simulink model "test"  (R2018b)
settings: Solver=VariableStepAuto  StartTime=0.0  StopTime=10  RelTol=1e-3
values from neighbouring files (symbols this model uses):
  A = jacobian([f1,f2, f3, f4], [x1, x2, x3, x4])    [TaylorRemainder.m]    (also in init_ctrl_design.m = eval(A); init_ctrl_design_simple.m = eval(A))
  Ad = expm(A*dT)    [init_ctrl_design.m]    (also in init_ctrl_design_simple.m = eye(2)+A*Ts)
  AK = Ad-Bd*K    [init_ctrl_design.m]    (also in init_ctrl_design_simple.m)
  B = jacobian([f1,f2, f3, f4], [u])    [TaylorRemainder.m]    (also in init_ctrl_design.m = eval(B); init_ctrl_design_simple.m = eval(B); mgcm_acado.m = 1)
  Bd = (Ad-eye(n))*inv(A)*B    [init_ctrl_design.m]    (also in init_ctrl_design_simple.m = Ts*B)
  beta = 1    [TaylorRemainder.m]    (also in init_ctrl_design.m; init_ctrl_design_simple.m; solveMGCM.m)
  C = eye(4)    [init_ctrl_design.m]    (also in init_ctrl_design_simple.m = eye(2))
  Cd = C    [init_ctrl_design.m]    (also in init_ctrl_design_simple.m = eye(2))
  D = zeros(4,1)    [init_ctrl_design.m]    (also in init_ctrl_design_simple.m = zeros(2,1))
  Dd = D    [init_ctrl_design.m]    (also in init_ctrl_design_simple.m)
  init_cond = [x1-0.35, x2-0.4, x3, 0]    [TaylorRemainder.m]    (also in init_ctrl_design.m; init_ctrl_design_simple.m = [x1-0.35, x2-0.4])
  Ts = 0.01    [APRBSgeneration.m]    (also in draw.m; drawCP.m = 0.1; genTrainingData.m = 0.1; init_ctrl_design.m)
  wn = sqrt(1000)    [TaylorRemainder.m]    (also in init_ctrl_design.m; solveMGCM.m)
  x2_c = 0    [TaylorRemainder.m]    (also in init_ctrl_design.m; init_ctrl_design_simple.m; solveMGCM.m)
  zeta = 1/sqrt(2)    [TaylorRemainder.m]    (also in init_ctrl_design.m)
undefined symbols (not defined in the file or in its folder): DiscIntNeverNeededParam, K
settings Model: Creator=pbevanda  LastModifiedBy=pbevanda

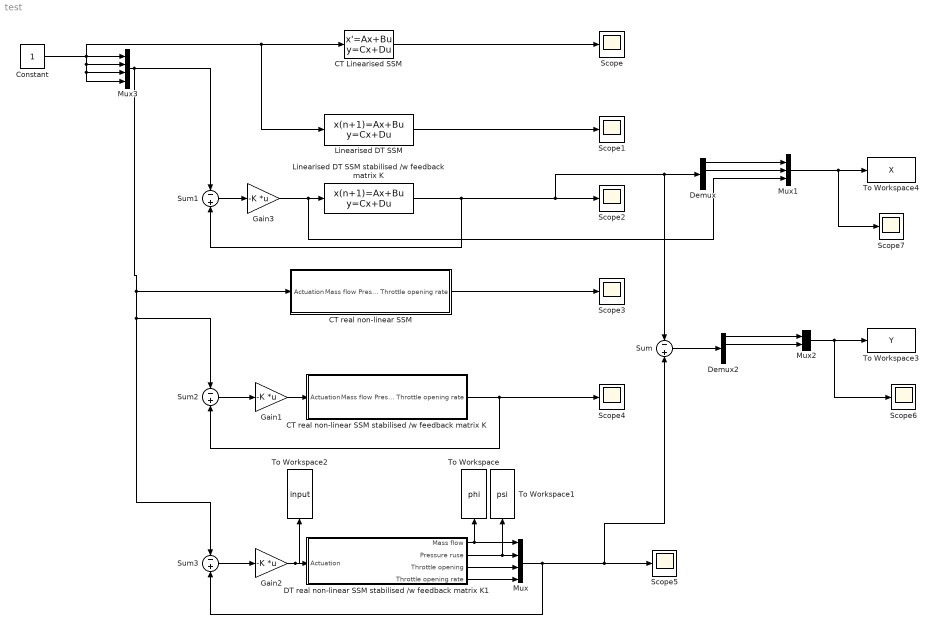
== system test ==
  CT Linearised SSM : StateSpace  A=A  B=B  C=C  D=D  InitialCondition=init_cond
  "CT real non-linear SSM " : Subsystem
  CT real non-linear SSM stabilised /w feedback matrix K : Subsystem
  Constant : Constant
  DT real non-linear SSM stabilised /w feedback matrix K1 : Subsystem
  Demux : Demux
  Demux2 : Demux
  Gain1 : Gain  Gain=-K  Multiplication=Matrix(K*u)
  Gain2 : Gain  Gain=-K  Multiplication=Matrix(K*u)
  Gain3 : Gain  Gain=-K  Multiplication=Matrix(K*u)
  "Linearised DT SSM " : DiscreteStateSpace  A=AK  B=Bd  C=Cd  D=Dd  InitialCondition=init_cond  SampleTime=Ts
  Linearised DT SSM stabilised /w feedback matrix K : DiscreteStateSpace  A=Ad  B=Bd  C=Cd  D=Dd  InitialCondition=init_cond  SampleTime=Ts
  Mux : Mux
  Mux1 : Mux  Inputs=3
  Mux2 : Mux  Inputs=2
  Mux3 : Mux
  Scope{,1..7} (8 alike) : Scope
  Sum{,1..3} (4 alike) : Sum  Inputs=-+
  To Workspace : ToWorkspace  VariableName=phi  SaveFormat=Timeseries  SampleTime=-1
  To Workspace1 : ToWorkspace  VariableName=psi  SaveFormat=Timeseries  SampleTime=-1
  To Workspace2 : ToWorkspace  VariableName=input  SaveFormat=Timeseries  SampleTime=-1
  To Workspace3 : ToWorkspace  VariableName=Y  SampleTime=-1
  To Workspace4 : ToWorkspace  VariableName=X  SampleTime=-1
  wires:
  Demux/2 -> Mux1/2
  CT Linearised SSM/1 -> Scope/1
  Mux/1 -> Sum3/2, Scope5/1, Sum/2
  "CT real non-linear SSM "/1("Mass flow Pressure ruse Throttle opening Throttle opening rate ") -> Scope3/1
  "Linearised DT SSM "/1 -> Scope1/1
  Gain3/1 -> Mux1/3, Linearised DT SSM stabilised /w feedback matrix K/1
  Sum/1 -> Demux2/1
  Sum1/1 -> Gain3/1
  DT real non-linear SSM stabilised /w feedback matrix K1/4("Throttle opening rate ") -> Mux/4
  DT real non-linear SSM stabilised /w feedback matrix K1/2("Pressure ruse ") -> To Workspace1/1, Mux/2
  Sum2/1 -> Gain1/1
  Constant/1 -> Mux3/1, Mux3/4, Mux3/3, Mux3/2, "Linearised DT SSM "/1, CT Linearised SSM/1
  Demux/1 -> Mux1/1
  DT real non-linear SSM stabilised /w feedback matrix K1/1("Mass flow ") -> To Workspace/1, Mux/1
  Linearised DT SSM stabilised /w feedback matrix K/1 -> Sum1/2, Sum/1, Demux/1, Scope2/1
  DT real non-linear SSM stabilised /w feedback matrix K1/3("Throttle opening ") -> Mux/3
  Sum3/1 -> Gain2/1
  Mux2/1 -> Scope6/1, To Workspace3/1
  Mux3/1 -> Sum1/1, Sum3/1, Sum2/1, "CT real non-linear SSM "/1("Actuation ")
  Demux2/1 -> Mux2/1
  Demux2/2 -> Mux2/2
  CT real non-linear SSM stabilised /w feedback matrix K/1("Mass flow Pressure ruse Throttle opening Throttle opening rate ") -> Sum2/2, Scope4/1
  Gain1/1 -> CT real non-linear SSM stabilised /w feedback matrix K/1("Actuation ")
  Gain2/1 -> To Workspace2/1, DT real non-linear SSM stabilised /w feedback matrix K1/1("Actuation ")
  Mux1/1 -> Scope7/1, To Workspace4/1

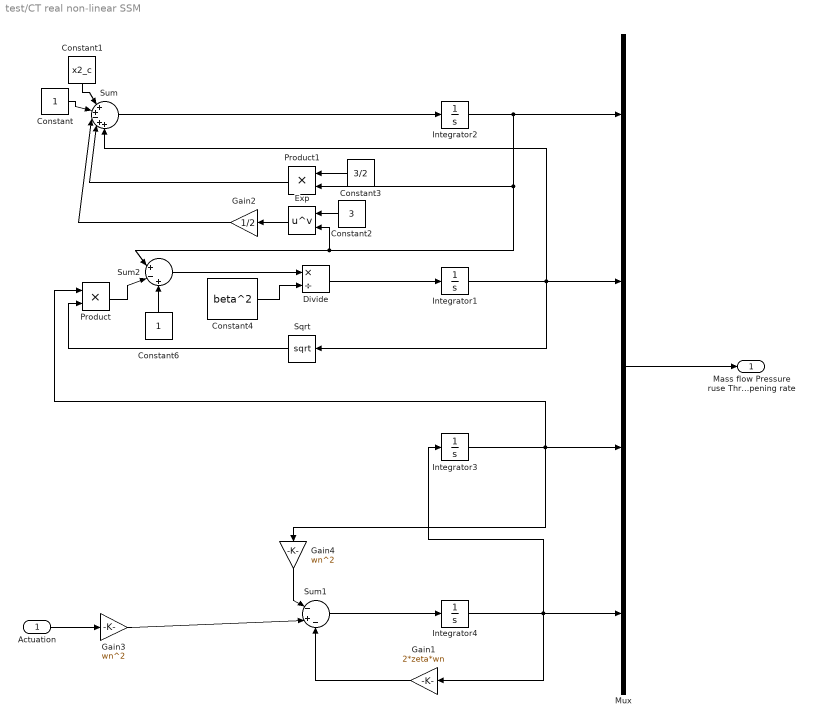
== system test/CT real non-linear SSM  ==
  "Actuation " : Inport
  Constant : Constant
  Constant1 : Constant  Value=x2_c
  Constant2 : Constant  Value=3
  Constant3 : Constant  Value=3/2
  Constant4 : Constant  Value=beta^2
  Constant6 : Constant
  Divide : Product  Inputs=*/
  Exp : Math  Operator=pow  SaturateOnIntegerOverflow=on
  Gain1 : Gain  Gain=2*zeta*wn
  Gain2 : Gain  Gain=1/2
  Gain3 : Gain  Gain=wn^2
  Gain4 : Gain  Gain=wn^2
  Integrator1 : Integrator  InitialCondition=init_cond(2)
  Integrator2 : Integrator  InitialCondition=init_cond(1)
  Integrator3 : Integrator  InitialCondition=init_cond(3)
  Integrator4 : Integrator  InitialCondition=init_cond(4)
  Mux : Mux
  Product : Product
  Product1 : Product
  Sqrt : Sqrt  SaturateOnIntegerOverflow=on
  Sum : Sum  Inputs=|++-++
  Sum1 : Sum  Inputs=|-+-
  Sum2 : Sum  Inputs=|+-+
  "Mass flow Pressure ruse Throttle opening Throttle opening rate " : Outport
  wires:
  Mux/1 -> "Mass flow Pressure ruse Throttle opening Throttle opening rate "/1
  Constant/1 -> Sum/2
  Constant1/1 -> Sum/1
  Constant2/1 -> Exp/1
  Constant4/1 -> Divide/2
  Sum2/1 -> Divide/1
  Integrator1/1 -> Sum/5, Mux/2, Sqrt/1
  Integrator2/1 -> Exp/2, Sum2/1, Product1/2, Mux/1
  Constant6/1 -> Sum2/3
  Sqrt/1 -> Product/2
  Product/1 -> Sum2/2
  Divide/1 -> Integrator1/1
  Exp/1 -> Gain2/1
  Gain2/1 -> Sum/3
  Sum/1 -> Integrator2/1
  Constant3/1 -> Product1/1
  Product1/1 -> Sum/4
  Integrator3/1 -> Gain4/1, Product/1, Mux/3
  Integrator4/1 -> Gain1/1, Integrator3/1, Mux/4
  "Actuation "/1 -> Gain3/1
  Sum1/1 -> Integrator4/1
  Gain1/1 -> Sum1/3
  Gain4/1 -> Sum1/1
  Gain3/1 -> Sum1/2

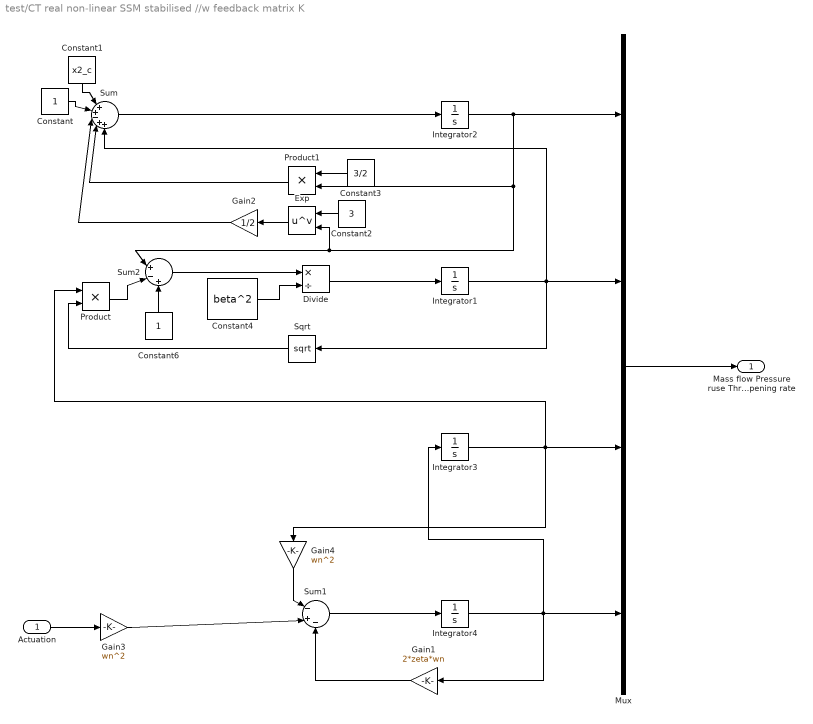
== system test/CT real non-linear SSM stabilised //w feedback matrix K ==
  "Actuation " : Inport
  Constant : Constant
  Constant1 : Constant  Value=x2_c
  Constant2 : Constant  Value=3
  Constant3 : Constant  Value=3/2
  Constant4 : Constant  Value=beta^2
  Constant6 : Constant
  Divide : Product  Inputs=*/
  Exp : Math  Operator=pow  SaturateOnIntegerOverflow=on
  Gain1 : Gain  Gain=2*zeta*wn
  Gain2 : Gain  Gain=1/2
  Gain3 : Gain  Gain=wn^2
  Gain4 : Gain  Gain=wn^2
  Integrator1 : Integrator  InitialCondition=init_cond(2)
  Integrator2 : Integrator  InitialCondition=init_cond(1)
  Integrator3 : Integrator  InitialCondition=init_cond(3)
  Integrator4 : Integrator  InitialCondition=init_cond(4)
  Mux : Mux
  Product : Product
  Product1 : Product
  Sqrt : Sqrt  SaturateOnIntegerOverflow=on
  Sum : Sum  Inputs=|++-++
  Sum1 : Sum  Inputs=|-+-
  Sum2 : Sum  Inputs=|+-+
  "Mass flow Pressure ruse Throttle opening Throttle opening rate " : Outport
  wires:
  Mux/1 -> "Mass flow Pressure ruse Throttle opening Throttle opening rate "/1
  Constant/1 -> Sum/2
  Constant1/1 -> Sum/1
  Constant2/1 -> Exp/1
  Constant4/1 -> Divide/2
  Sum2/1 -> Divide/1
  Integrator1/1 -> Sum/5, Mux/2, Sqrt/1
  Integrator2/1 -> Exp/2, Sum2/1, Product1/2, Mux/1
  Constant6/1 -> Sum2/3
  Sqrt/1 -> Product/2
  Product/1 -> Sum2/2
  Divide/1 -> Integrator1/1
  Exp/1 -> Gain2/1
  Gain2/1 -> Sum/3
  Sum/1 -> Integrator2/1
  Constant3/1 -> Product1/1
  Product1/1 -> Sum/4
  Integrator3/1 -> Gain4/1, Product/1, Mux/3
  Integrator4/1 -> Gain1/1, Integrator3/1, Mux/4
  "Actuation "/1 -> Gain3/1
  Sum1/1 -> Integrator4/1
  Gain1/1 -> Sum1/3
  Gain4/1 -> Sum1/1
  Gain3/1 -> Sum1/2

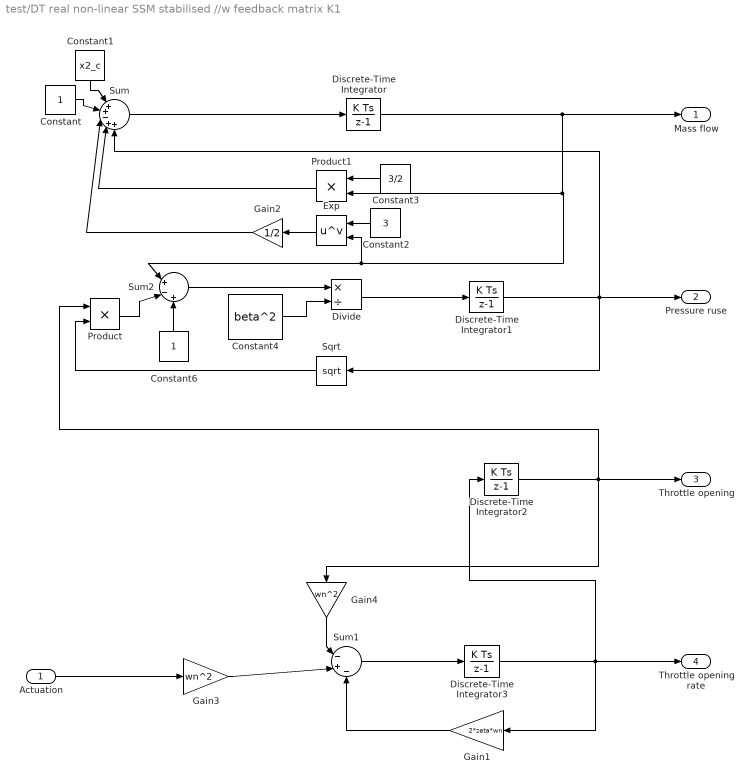
== system test/DT real non-linear SSM stabilised //w feedback matrix K1 ==
  "Actuation " : Inport
  Constant : Constant
  Constant1 : Constant  Value=x2_c
  Constant2 : Constant  Value=3
  Constant3 : Constant  Value=3/2
  Constant4 : Constant  Value=beta^2
  Constant6 : Constant
  Discrete-Time Integrator : DiscreteIntegrator  InitialCondition=init_cond(1)  SampleTime=-1  ICPrevOutput=DiscIntNeverNeededParam  ICPrevScaledInput=DiscIntNeverNeededParam
  Discrete-Time Integrator1 : DiscreteIntegrator  InitialCondition=init_cond(2)  SampleTime=-1  ICPrevOutput=DiscIntNeverNeededParam  ICPrevScaledInput=DiscIntNeverNeededParam
  Discrete-Time Integrator2 : DiscreteIntegrator  InitialCondition=init_cond(3)  SampleTime=-1  ICPrevOutput=DiscIntNeverNeededParam  ICPrevScaledInput=DiscIntNeverNeededParam
  Discrete-Time Integrator3 : DiscreteIntegrator  InitialCondition=init_cond(4)  SampleTime=-1  ICPrevOutput=DiscIntNeverNeededParam  ICPrevScaledInput=DiscIntNeverNeededParam
  Divide : Product  Inputs=*/
  Exp : Math  Operator=pow  SaturateOnIntegerOverflow=on
  Gain1 : Gain  Gain=2*zeta*wn
  Gain2 : Gain  Gain=1/2
  Gain3 : Gain  Gain=wn^2
  Gain4 : Gain  Gain=wn^2
  Product : Product
  Product1 : Product
  Sqrt : Sqrt  SaturateOnIntegerOverflow=on
  Sum : Sum  Inputs=|++-++
  Sum1 : Sum  Inputs=|-+-
  Sum2 : Sum  Inputs=|+-+
  "Mass flow " : Outport
  "Pressure ruse " : Outport  Port=2
  "Throttle opening " : Outport  Port=3
  "Throttle opening rate " : Outport  Port=4
  wires:
  Constant/1 -> Sum/2
  Constant1/1 -> Sum/1
  Constant2/1 -> Exp/1
  Constant4/1 -> Divide/2
  Sum2/1 -> Divide/1
  Constant6/1 -> Sum2/3
  Sqrt/1 -> Product/2
  Product/1 -> Sum2/2
  Divide/1 -> Discrete-Time Integrator1/1
  Exp/1 -> Gain2/1
  Gain2/1 -> Sum/3
  Constant3/1 -> Product1/1
  Product1/1 -> Sum/4
  Sum1/1 -> Discrete-Time Integrator3/1
  Gain1/1 -> Sum1/3
  Gain4/1 -> Sum1/1
  Sum/1 -> Discrete-Time Integrator/1
  Gain3/1 -> Sum1/2
  "Actuation "/1 -> Gain3/1
  Discrete-Time Integrator2/1 -> "Throttle opening "/1, Gain4/1, Product/1
  Discrete-Time Integrator3/1 -> "Throttle opening rate "/1, Discrete-Time Integrator2/1, Gain1/1
  Discrete-Time Integrator/1 -> "Mass flow "/1, Product1/2, Exp/2, Sum2/1
  Discrete-Time Integrator1/1 -> "Pressure ruse "/1, Sum/5, Sqrt/1
